simulink model "Trapezi_Ergasias_24_Scenario_1"  (R2023a)
settings: Solver=VariableStepAuto  StartTime=0.0  StopTime=10.0  RelTol=1e-3
libraries: fuzblock x1
settings Model: Creator=User  LastModifiedBy=User
settings DebuggingCC: UnconnectedInputMsg=warning  UnconnectedOutputMsg=warning  UnconnectedLineMsg=warning
settings ModelReferenceCC: EnableRefExpFcnMdlSchedulingChecks=on
settings RTWCC: DLArmComputeVersion=19.05

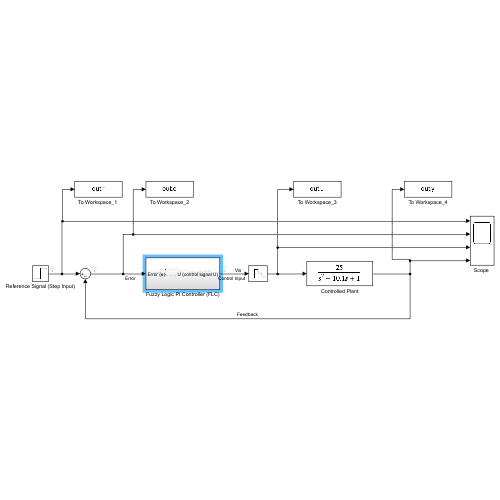
[thumbnail: Simulink's stored preview of the top-level diagram]
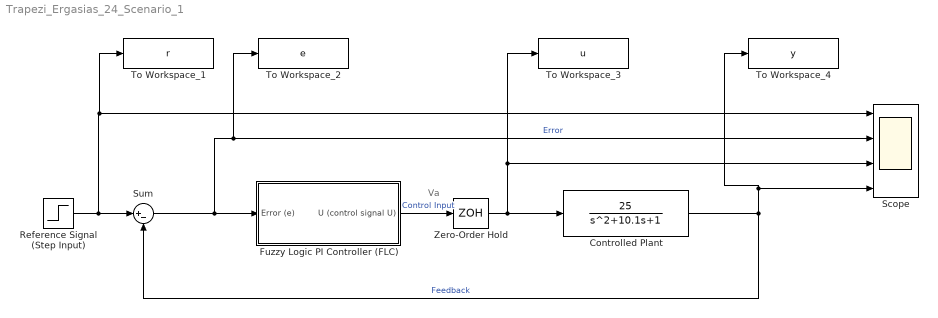
== system Trapezi_Ergasias_24_Scenario_1 ==
  note: Va
  Controlled Plant : TransferFcn  Numerator=[25]  Denominator=[1 10.1 1]
  Fuzzy Logic PI Controller (FLC) : Subsystem
  Reference Signal (Step Input) : Step  After=50  SampleTime=0
  "Scope " : Scope  NumInputPorts=4
  Sum : Sum  Inputs=|+-
  "To Workspace_1 " : ToWorkspace  VariableName=r  SaveFormat=Timeseries  SampleTime=-1
  To Workspace_2 : ToWorkspace  VariableName=e  SaveFormat=Timeseries  SampleTime=-1
  To Workspace_3 : ToWorkspace  VariableName=u  SaveFormat=Timeseries  SampleTime=-1
  To Workspace_4 : ToWorkspace  VariableName=y  SaveFormat=Timeseries  SampleTime=-1
  Zero-Order Hold : ZeroOrderHold  SampleTime=-1
  wires:
  Reference Signal (Step Input)/1 -> "To Workspace_1 "/1, "Scope "/1, Sum/1
  Controlled Plant/1 -> To Workspace_4/1, "Scope "/4, Sum/2  "Feedback"
  Sum/1 -> Fuzzy Logic PI Controller (FLC)/1(Error (e)), To Workspace_2/1, "Scope "/2  "Error"
  Fuzzy Logic PI Controller (FLC)/1("\tU (control signal U)") -> Zero-Order Hold/1  "Control Input"
  Zero-Order Hold/1 -> To Workspace_3/1, "Scope "/3, Controlled Plant/1

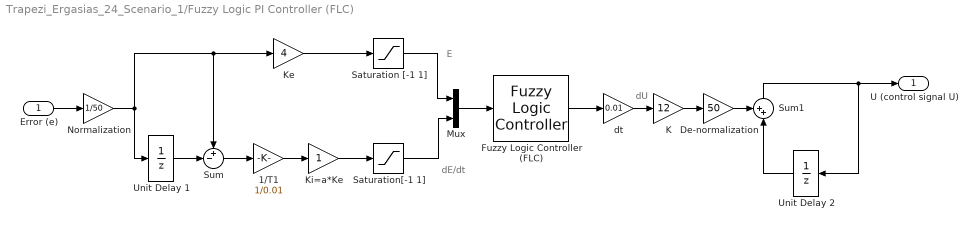
== system Trapezi_Ergasias_24_Scenario_1/Fuzzy Logic PI Controller (FLC) ==
  note: dU
  note: E
  note: dE/dt
  Error (e) : Inport
  1/Τ1 : Gain  Gain=1/0.01
  De-normalization : Gain  Gain=50
  Fuzzy Logic Controller (FLC) : fuzblock/Fuzzy Logic  Controller  FIS='FISystem_Trapezi_Ergasias_24.fis'  OutputSampleNumber=101  DataType=double  FuzzifiedInputs=off  RuleFiringStrengths=off  RuleOutputs=off  AggregatedOutputs=off  SimulateUsing=Interpreted execution  OutOfRangeInputValueMessage=warning  NoRuleFiredMessage=warning  EmptyOutputFuzzySetMessage=warning
  K : Gain  Gain=12
  Ke : Gain  Gain=4
  Ki=a*Ke : Gain
  Mux : Mux  Inputs=2
  Normalization : Gain  Gain=1/50
  Saturation [-1 1] : Saturate  UpperLimit=1  LowerLimit=-1
  "Saturation[-1 1] " : Saturate  UpperLimit=1  LowerLimit=-1
  Sum : Sum  Inputs=+-|
  Sum1 : Sum  Inputs=++|
  Unit Delay 1 : UnitDelay  SampleTime=0.01  HasFrameUpgradeWarning=on
  Unit Delay 2 : UnitDelay  SampleTime=0.01  HasFrameUpgradeWarning=on
  dt : Gain  Gain=0.01
  "\tU (control signal U)" : Outport
  wires:
  Error (e)/1 -> Normalization/1
  Fuzzy Logic Controller (FLC)/1 -> dt/1
  Mux/1 -> Fuzzy Logic Controller (FLC)/1
  1/Τ1/1 -> Ki=a*Ke/1
  Ke/1 -> Saturation [-1 1]/1
  Normalization/1 -> Unit Delay 1/1, Ke/1, Sum/1
  Saturation [-1 1]/1 -> Mux/1
  "Saturation[-1 1] "/1 -> Mux/2
  Unit Delay 1/1 -> Sum/2
  Sum/1 -> 1/Τ1/1
  De-normalization/1 -> Sum1/1
  Unit Delay 2/1 -> Sum1/2
  Ki=a*Ke/1 -> "Saturation[-1 1] "/1
  dt/1 -> K/1
  K/1 -> De-normalization/1
  Sum1/1 -> Unit Delay 2/1, "\tU (control signal U)"/1
